simulink model "TPLIA_Input"  (R2020b)
settings: Solver=VariableStepAuto  StartTime=0.0  StopTime=500  FixedStep=0.000001  MaxStep=1e-4  RelTol=1e-3  EnableMultiTasking=on
libraries: dspsrcs4 x3, dspfdesign x2, simulink x1
settings Model: Creator=LYX  LastModifiedBy=LYX
settings OptimizationCC: DefaultUnderspecifiedDataType=single

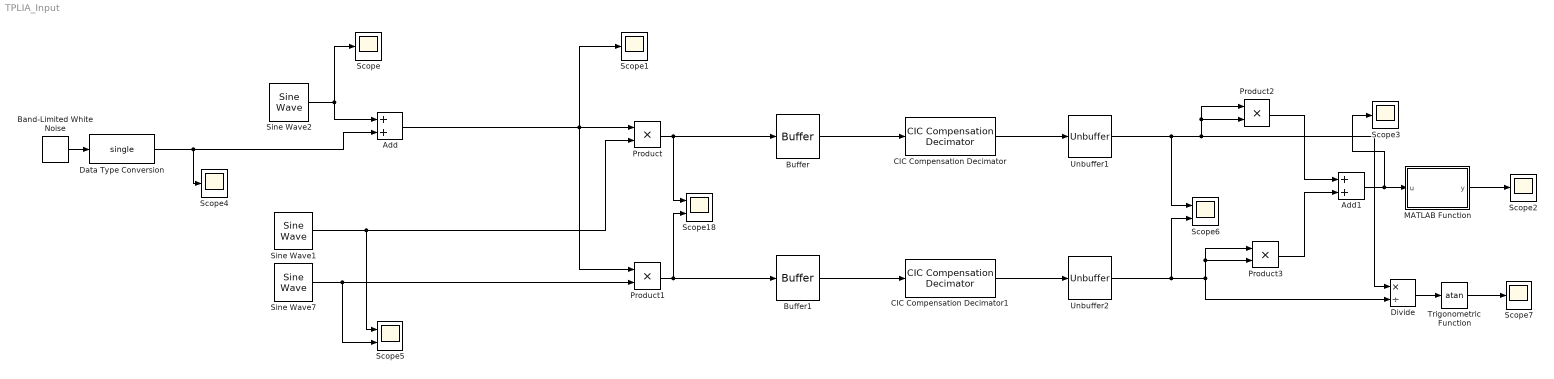
== system TPLIA_Input ==
  Add : Sum
  Add1 : Sum
  Band-Limited White Noise : simulink/Sources/Band-Limited White Noise  Cov=[0.00001*0.00001*0.01]  Ts=0.1  seed=[23341]
  Buffer : Buffer  N=8  OutputFrames=off
  Buffer1 : Buffer  N=8  OutputFrames=off
  CIC Compensation Decimator : dspfdesign/CIC Compensation Decimator  CICRateChangeFactor=4  CICNumSections=8  CICDifferentialDelay=1  DecimationFactor=4  DesignForMinimumOrder=on  FilterOrder=12  PassbandFrequency=0.2  StopbandFrequency=10  PassbandRipple=1  StopbandAttenuation=90  InheritSampleRate=on  SampleRate=960  SimulateUsing=Code generation  roundingMode=Floor  coeffsDataTypeStr=fixdt(1,16)
      settings: SourceProductBaseCode=DS
  CIC Compensation Decimator1 : dspfdesign/CIC Compensation Decimator  CICRateChangeFactor=4  CICNumSections=8  CICDifferentialDelay=1  DecimationFactor=4  DesignForMinimumOrder=on  FilterOrder=12  PassbandFrequency=0.2  StopbandFrequency=10  PassbandRipple=1  StopbandAttenuation=90  InheritSampleRate=on  SampleRate=1200000  SimulateUsing=Code generation  roundingMode=Floor  coeffsDataTypeStr=fixdt(1,16)
      settings: SourceProductBaseCode=DS
  Data Type Conversion : DataTypeConversion  OutDataTypeStr=single
  Divide : Product  Inputs=*/
  MATLAB Function : MATLAB Function  TreatAsAtomicUnit=on
  Product{,1..3} (4 alike) : Product
  Scope{,1..4,7} (6 alike) : Scope
  Scope18 : Scope  NumInputPorts=2
  Scope5 : Scope  NumInputPorts=2
  Scope6 : Scope  NumInputPorts=2
  Sine Wave1 : dspsrcs4/Sine Wave  Amplitude=1  Frequency=20  Phase=0  SampleMode=Discrete  OutComplex=Real  CompMethod=Trigonometric fcn  TableSize=Speed  SampleTime=1/960  SamplesPerFrame=1  ResetState=Restart at time zero  OutputFrames=off  dataType=single  wordLen=16  udDataType=sfix(16)  fracBitsMode=Best precision  numFracBits=15  OutDataTypeStr=single  LastOutDataTypeStr=single
  Sine Wave2 : dspsrcs4/Sine Wave  Amplitude=0.01  Frequency=20  Phase=0  SampleMode=Discrete  OutComplex=Real  CompMethod=Trigonometric fcn  TableSize=Speed  SampleTime=1/960  SamplesPerFrame=1  ResetState=Restart at time zero  OutputFrames=off  dataType=single  wordLen=16  udDataType=sfix(16)  fracBitsMode=Best precision  numFracBits=15  OutDataTypeStr=single  LastOutDataTypeStr=single
  Sine Wave7 : dspsrcs4/Sine Wave  Amplitude=1  Frequency=20  Phase=pi/2  SampleMode=Discrete  OutComplex=Real  CompMethod=Trigonometric fcn  TableSize=Speed  SampleTime=1/960  SamplesPerFrame=1  ResetState=Restart at time zero  OutputFrames=off  dataType=single  wordLen=16  udDataType=sfix(16)  fracBitsMode=Best precision  numFracBits=15  OutDataTypeStr=single  LastOutDataTypeStr=single
  Trigonometric Function : Trigonometry  Operator=atan
  Unbuffer1 : Unbuffer
  Unbuffer2 : Unbuffer
  wires:
  Sine Wave2/1 -> Add/1, Scope/1
  Sine Wave1/1 -> Scope5/1, Product/2
  Sine Wave7/1 -> Scope5/2, Product1/2
  Product2/1 -> Add1/1
  Product3/1 -> Add1/2
  Add1/1 -> Scope3/1, MATLAB Function/1(u)
  MATLAB Function/1(y) -> Scope2/1
  Divide/1 -> Trigonometric Function/1
  Trigonometric Function/1 -> Scope7/1
  Unbuffer1/1 -> Scope6/1, Divide/1, Product2/2, Product2/1
  Unbuffer2/1 -> Scope6/2, Divide/2, Product3/2, Product3/1
  CIC Compensation Decimator/1 -> Unbuffer1/1
  CIC Compensation Decimator1/1 -> Unbuffer2/1
  Product/1 -> Buffer/1, Scope18/1
  Product1/1 -> Buffer1/1, Scope18/2
  Buffer/1 -> CIC Compensation Decimator/1
  Buffer1/1 -> CIC Compensation Decimator1/1
  Add/1 -> Product1/1, Scope1/1, Product/1
  Band-Limited White Noise/1 -> Data Type Conversion/1
  Data Type Conversion/1 -> Scope4/1, Add/2

== matlab function TPLIA_Input/MATLAB Function ==
  data: u input; y output
function y = fcn(u)

y = 2 * sqrt(u);
